simulink library "asbhl20GPS"  (R2016b)
settings: Solver=VariableStepAuto  StartTime=0.0  StopTime=10.0  RelTol=1e-3
undefined symbols (not defined in the file): Tc
libraries: aerolibconvert2 x1, aerolibtransform2 x1
Description:
  | HL-20 Global Positioning System (GPS) receiver component model
settings Model: Creator=The MathWorks, Inc.  LastModifiedBy=The MathWorks, Inc.
settings DataIOCC: LimitDataPoints=on  SaveFormat=Array  SignalLoggingSaveFormat=ModelDataLogs
settings OptimizationCC: BlockReduction=off  BooleanDataType=off  LifeSpan=inf
settings DebuggingCC: SaveWithParameterizedLinksMsg=none  UnderspecifiedInitializationDetection=Classic  MergeDetectMultiDrivingBlocksExec=none  SignalResolutionControl=TryResolveAllWithWarning  AllowSymbolicDim=off  StrictBusMsg=Warning  SFUnexpectedBacktrackingDiag=warning  SFNoUnconditionalDefaultTransitionDiag=warning  SFExecutionAtInitializationDiag=none
settings HardwareCC: ProdBitPerPointer=32  ProdBitPerSizeT=32  ProdBitPerPtrDiffT=32  ProdLargestAtomicFloat=None  ProdIntDivRoundTo=Undefined  ProdEndianess=Unspecified  ProdWordSize=32  ProdHWDeviceType=32-bit Generic  TargetUnknown=on
settings ModelReferenceCC: PropagateSignalLabelsOutOfModel=off
settings GRTTargetCC: TargetLangStandard=C89/C90 (ANSI)
settings ConfigComp: CovMetricSettings=dw  CovHtmlReporting=on  CovSaveCumulativeToWorkspaceVar=on  CovSaveSingleToWorkspaceVar=on  CovExternalEMLEnable=off

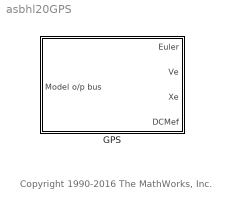
== system asbhl20GPS ==
  note: Copyright 1990-2016 The MathWorks, Inc.
  GPS : Subsystem  TreatAsAtomicUnit=on

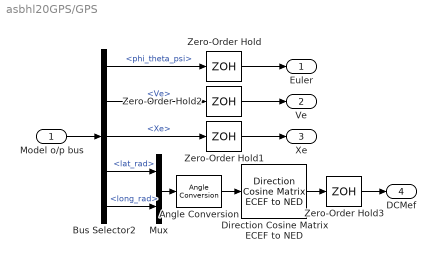
== system asbhl20GPS/GPS ==
  Model o/p bus : Inport
  Angle Conversion : aerolibconvert2/Angle Conversion  IU=rad  OU=deg
  Bus Selector2 : BusSelector  OutputSignals=phi_theta_psi,Ve,Xe,PosLLA.lat_rad,PosLLA.long_rad
  Direction Cosine Matrix ECEF to NED : aerolibtransform2/Direction Cosine Matrix ECEF to NED
  Mux : Mux  Inputs=2
  Zero-Order Hold{,1..3} (4 alike) : ZeroOrderHold  SampleTime=Tc
  Euler : Outport  Unit=rad
  Ve : Outport  Port=2  Unit=m/s
  Xe : Outport  Port=3  Unit=m
  DCMef : Outport  Port=4
  wires:
  Bus Selector2/5 -> Mux/2  "<long_rad>"
  Bus Selector2/4 -> Mux/1  "<lat_rad>"
  Mux/1 -> Angle Conversion/1
  Zero-Order Hold3/1 -> DCMef/1
  Direction Cosine Matrix ECEF to NED/1 -> Zero-Order Hold3/1
  Model o/p bus/1 -> Bus Selector2/1
  Bus Selector2/3 -> Zero-Order Hold1/1  "<Xe>"
  Zero-Order Hold/1 -> Euler/1
  Zero-Order Hold1/1 -> Xe/1
  Bus Selector2/1 -> Zero-Order Hold/1  "<phi_theta_psi>"
  Bus Selector2/2 -> Zero-Order Hold2/1  "<Ve>"
  Zero-Order Hold2/1 -> Ve/1
  Angle Conversion/1 -> Direction Cosine Matrix ECEF to NED/1
